simulink model "inverted_pendulum_2D"  (R2016a)
settings: Solver=ode5  SolverMode=SingleTasking  StartTime=0.0  StopTime=Inf  FixedStep=0.01  MaxStep=0.02  RelTol=1e-3
undefined symbols (not defined in the file or in its folder): sl3d_sfuntraj
libraries: vrlib x1
Description:
  | Inverted Pendulum
  | 
  | The vrpend example illustrates the various ways a dynamic model in Simulink(R) can
  | interact with a virtual reality world. It is the model of 2-dimensional inverted pendulum
  | controlled by a PID controller. What distinguishes this model from 'common' inverted
  | pendulum models is visualization and the methods of setting the setpoint. You visualize
  | and interact with a virtual world by using a Trajectory Graph and VR Sink blocks.
  | The Trajectory Graph block allows you to track the history of the pendulum position
  | and change the setpoint. The method for setting the setpoint can be selected in
  | the mask of the Trajectory Graph block. The following methods are available:
  | 
  |   Mouse - Click-and-drag a mouse pointer in the Trajectory Graph 2-D window
  | 
  |   Input Signal - External Trajectory Graph input in this model driven by a random number generator
  | 
  |   VR Sensor - Activates the input from a VRML TouchSensor
  | 
  | When the pointing device in the VRML viewer moves over an active TouchSensor area,
  | the cursor shape changes from an arrow to a hand shape. When the setpoint selection method
  | is set to VRSensor, left mouse button click sets the new setpoint value.
  | 
  | Notice the pseudo orthographic view defined in the associated VRML file. This effect is
  | achieved by creating a viewpoint which is located far from the object of interest with a very narrow
  | view defined by the VRML FieldOfView parameter. An orthographic view is useful for eliminating
  | the panoramic distortion that occurs when using a wide-angle lens. This technique is also
  | known in photography. The fallback of this technique is that locating the viewpoint in a distance
  | makes the standard viewer navigation tricky or difficult in some navigation modes. If you want
  | to navigate around the virtual pendulum bench, we recommend that you switch to some other viewpoint.
settings Model: FPTRunName=Active  ExtModeTrigDuration=100  Creator=The MathWorks, Inc.  LastModifiedBy=USER
settings DataIOCC: LimitDataPoints=on  SaveFormat=Array  SaveOutput=off  SaveTime=off  SignalLoggingName=logsOut
settings OptimizationCC: BlockReduction=off  BooleanDataType=off  ExpressionDepthLimit=2147483647  InitFltsAndDblsToZero=on
settings DebuggingCC: UnderspecifiedInitializationDetection=Classic  MergeDetectMultiDrivingBlocksExec=none  CheckExecutionContextPreStartOutputMsg=on  CheckExecutionContextRuntimeOutputMsg=on  SignalResolutionControl=TryResolveAllWithWarning  MultiTaskDSMMsg=warning  MultiTaskCondExecSysMsg=none  FcnCallInpInsideContextMsg=UseLocalSettings  StateNameClashWarn=warning
settings HardwareCC: ProdBitPerPointer=32  ProdLargestAtomicFloat=None  ProdIntDivRoundTo=Undefined  ProdEndianess=Unspecified  ProdWordSize=32  ProdHWDeviceType=32-bit Generic  TargetUnknown=on
settings ModelReferenceCC: UpdateModelReferenceTargets=IfOutOfDate  PropagateSignalLabelsOutOfModel=off
settings GRTTargetCC: TargetFcnLib=ansi_tfl_tmw.mat  CombineOutputUpdateFcns=off  GRTInterface=on
settings ConfigComp: CovMetricSettings=d  CovModelRefEnable=Off  CovSFcnEnable=off

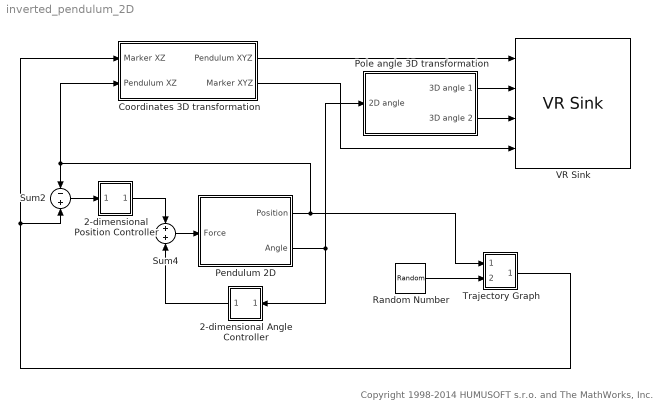
== system inverted_pendulum_2D ==
  note: Copyright 1998-2014 HUMUSOFT s.r.o. and The MathWorks, Inc.
  2-dimensional Angle Controller : Subsystem  mask(PID Controller){P=83.2, I=38.3, D=27.3}
      mask prompts: P "Proportional:"; I "Integral:"; D "Derivative:"
      mask help:
      | Enter expressions for proportional, integral, and derivative terms.
      | P+I/s+Ds
      mask Help: This block implements a PID controller where parameters are entered for the Proportional, Integral and Derivative terms. Unmask this block to see how it works. The derivative term is implemented using a true derivative block.
      mask Display: disp('PID')
  2-dimensional Position Controller : Subsystem  mask(PID Controller){P=-1.681, I=-0.0133, D=-0.325}
      mask prompts: P "Proportional:"; I "Integral:"; D "Derivative:"
      mask help:
      | Enter expressions for proportional, integral, and derivative terms.
      | P+I/s+Ds
      mask Help: This block implements a PID controller where parameters are entered for the Proportional, Integral and Derivative terms. Unmask this block to see how it works. The derivative term is implemented using a true derivative block.
      mask Display: disp('PID')
  Coordinates 3D transformation : Subsystem
  Pendulum 2D : Subsystem  mask(Inverted pendulum){mc=0.5, mp=1, l=0.5, g=9.80665}
      mask prompts: mc "Mass of cart (kg):"; mp "Mass of pendulum (kg):"; l "Distance to pendulum center of mass(m):"; g "Acceleration of gravity (m/s^2):"
      mask help: Look under mask to see dynamics
      mask Help: Nonlinear dynamics of inverted pendulum.
      mask Display: plot([-10 10],[0 0],[-2 -2 2 2],[0 1 1 0],[0 -2],[1 5])
  Pole angle 3D transformation : Subsystem
  Random Number : RandomNumber  Mean=[0 0]  Variance=[5 5]  Seed=[0 5]  SampleTime=3
  Sum2 : Sum  Inputs=-+  SaturateOnIntegerOverflow=on  InputSameDT=on  OutDataTypeStr=Inherit: Same as first input
  Sum4 : Sum  SaturateOnIntegerOverflow=on  InputSameDT=on  OutDataTypeStr=Inherit: Same as first input
  Trajectory Graph : Subsystem  LoadFcn=sl3d_sfuntraj([],[],[],'LoadBlock')  StartFcn=sl3d_sfuntraj([],[],[],'Start')  StopFcn=sl3d_sfuntraj([],[],[],'Stop')  TreatAsAtomicUnit=on  mask(Trajectory scope.){xmin=-10, xmax=10, ymin=-10, ymax=10, Ts=0.2, mode=VR sensor}
      mask prompts: xmin "x-min:"; xmax "x-max:"; ymin "y-min:"; ymax "y-max:"; Ts "Sample time:"; mode "Setpoint mode"
      mask help: Trajectory scope using MATLAB graph window. Enter plotting ranges.
      settings: CopyFcn=sl3d_sfuntraj([],[],[],'CopyBlock')  DeleteFcn=sl3d_sfuntraj([],[],[],'DeleteBlock')  NameChangeFcn=sl3d_sfuntraj([],[],[],'NameChange')
      mask Help: Look at the MATLAB function sl3d_sfuntraj.m to see how this block works.
      mask TypeOptions mode: Mouse | Input signal | VR sensor
      mask Display: plot([.05 .95 .95 .05 .05],[.45 .45 .95 .95 .45], 0.5+cos(0:0.1:2*pi)*0.3,0.7+sin(0:0.1:2*pi)*0.2)
  VR Sink : vrlib/VR Sink  InstantiateOnLoad=on  SampleTime=0.2  ViewEnable=on  RemoteChange=off  RemoteView=off  FieldsWritten=Pendulum.translation.3.1.1.double#Pole1.rotation.4.1.1.double#Pole2.rotation.4.1.1.double#Marker.translation.3.1.1.double  WorldFileName=vrpend.wrl  WorldDescription=Inverted Pendulum  AutoView=on  VideoDimensions=[]  AllowVariableSize=off
  wires:
  Sum4/1 -> Pendulum 2D/1(Force)
  2-dimensional Angle Controller/1(Out_1) -> Sum4/2
  2-dimensional Position Controller/1(Out_1) -> Sum4/1
  Sum2/1 -> 2-dimensional Position Controller/1(In_1)
  Pendulum 2D/2(Angle) -> 2-dimensional Angle Controller/1(In_1), Pole angle 3D transformation/1(2D angle)
  Pendulum 2D/1(Position) -> Sum2/1, Coordinates 3D transformation/2(Pendulum XZ), Trajectory Graph/1(data)
  Trajectory Graph/1(mouse) -> Sum2/2, Coordinates 3D transformation/1(Marker XZ)
  Random Number/1 -> Trajectory Graph/2(setpoint)
  Coordinates 3D transformation/2(Marker XYZ) -> VR Sink/4
  Coordinates 3D transformation/1(Pendulum XYZ) -> VR Sink/1
  Pole angle 3D transformation/1(3D angle 1) -> VR Sink/2
  Pole angle 3D transformation/2(3D angle 2) -> VR Sink/3

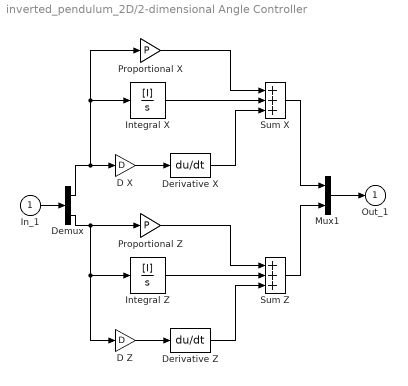
== system inverted_pendulum_2D/2-dimensional Angle Controller ==
  In_1 : Inport
  D X : Gain  Gain=D  SaturateOnIntegerOverflow=on  OutDataTypeStr=Inherit: Same as input  ParamDataTypeStr=Inherit: Same as input
  D Z : Gain  Gain=D  SaturateOnIntegerOverflow=on  OutDataTypeStr=Inherit: Same as input  ParamDataTypeStr=Inherit: Same as input
  Demux : Demux  Outputs=2
  Derivative X : Derivative
  Derivative Z : Derivative
  Integral X : TransferFcn  Numerator=[I]  Denominator=[1 0]
  Integral Z : TransferFcn  Numerator=[I]  Denominator=[1 0]
  Mux1 : Mux  Inputs=2
  Proportional X : Gain  Gain=P  SaturateOnIntegerOverflow=on  OutDataTypeStr=Inherit: Same as input  ParamDataTypeStr=Inherit: Same as input
  Proportional Z : Gain  Gain=P  SaturateOnIntegerOverflow=on  OutDataTypeStr=Inherit: Same as input  ParamDataTypeStr=Inherit: Same as input
  Sum X : Sum  Inputs=+++  SaturateOnIntegerOverflow=on  InputSameDT=on  OutDataTypeStr=Inherit: Same as first input
  Sum Z : Sum  Inputs=+++  SaturateOnIntegerOverflow=on  InputSameDT=on  OutDataTypeStr=Inherit: Same as first input
  Out_1 : Outport  InitialOutput=0
  wires:
  D X/1 -> Derivative X/1
  Derivative X/1 -> Sum X/3
  Integral X/1 -> Sum X/2
  Proportional X/1 -> Sum X/1
  In_1/1 -> Demux/1
  Demux/2 -> Proportional Z/1, Integral Z/1, D Z/1
  Demux/1 -> D X/1, Integral X/1, Proportional X/1
  Sum X/1 -> Mux1/1
  Sum Z/1 -> Mux1/2
  D Z/1 -> Derivative Z/1
  Derivative Z/1 -> Sum Z/3
  Integral Z/1 -> Sum Z/2
  Proportional Z/1 -> Sum Z/1
  Mux1/1 -> Out_1/1

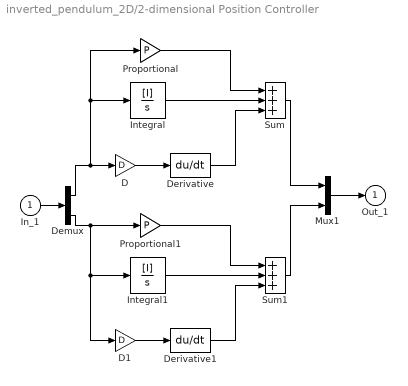
== system inverted_pendulum_2D/2-dimensional Position Controller ==
  In_1 : Inport
  D : Gain  Gain=D  SaturateOnIntegerOverflow=on  OutDataTypeStr=Inherit: Same as input  ParamDataTypeStr=Inherit: Same as input
  D1 : Gain  Gain=D  SaturateOnIntegerOverflow=on  OutDataTypeStr=Inherit: Same as input  ParamDataTypeStr=Inherit: Same as input
  Demux : Demux  Outputs=2
  Derivative : Derivative
  Derivative1 : Derivative
  Integral : TransferFcn  Numerator=[I]  Denominator=[1 0]
  Integral1 : TransferFcn  Numerator=[I]  Denominator=[1 0]
  Mux1 : Mux  Inputs=2
  Proportional : Gain  Gain=P  SaturateOnIntegerOverflow=on  OutDataTypeStr=Inherit: Same as input  ParamDataTypeStr=Inherit: Same as input
  Proportional1 : Gain  Gain=P  SaturateOnIntegerOverflow=on  OutDataTypeStr=Inherit: Same as input  ParamDataTypeStr=Inherit: Same as input
  Sum : Sum  Inputs=+++  SaturateOnIntegerOverflow=on  InputSameDT=on  OutDataTypeStr=Inherit: Same as first input
  Sum1 : Sum  Inputs=+++  SaturateOnIntegerOverflow=on  InputSameDT=on  OutDataTypeStr=Inherit: Same as first input
  Out_1 : Outport  InitialOutput=0
  wires:
  Mux1/1 -> Out_1/1
  Proportional1/1 -> Sum1/1
  Integral1/1 -> Sum1/2
  Derivative1/1 -> Sum1/3
  D1/1 -> Derivative1/1
  Sum1/1 -> Mux1/2
  Sum/1 -> Mux1/1
  Demux/1 -> Proportional/1, Integral/1, D/1
  Demux/2 -> D1/1, Integral1/1, Proportional1/1
  In_1/1 -> Demux/1
  Proportional/1 -> Sum/1
  Integral/1 -> Sum/2
  Derivative/1 -> Sum/3
  D/1 -> Derivative/1

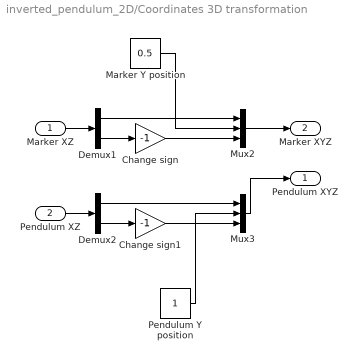
== system inverted_pendulum_2D/Coordinates 3D transformation ==
  Marker XZ : Inport
  Pendulum XZ : Inport  Port=2
  Change sign : Gain  Gain=-1
  Change sign1 : Gain  Gain=-1
  Demux1 : Demux  Outputs=2
  Demux2 : Demux  Outputs=2
  Marker Y position : Constant  Value=0.5
  Mux2 : Mux  Inputs=3
  Mux3 : Mux  Inputs=3
  Pendulum Y position : Constant
  Pendulum XYZ : Outport
  Marker XYZ : Outport  Port=2
  wires:
  Marker XZ/1 -> Demux1/1
  Pendulum XZ/1 -> Demux2/1
  Pendulum Y position/1 -> Mux3/2
  Marker Y position/1 -> Mux2/2
  Mux2/1 -> Marker XYZ/1
  Mux3/1 -> Pendulum XYZ/1
  Demux1/1 -> Mux2/1
  Demux1/2 -> Change sign/1
  Demux2/2 -> Change sign1/1
  Change sign/1 -> Mux2/3
  Demux2/1 -> Mux3/1
  Change sign1/1 -> Mux3/3

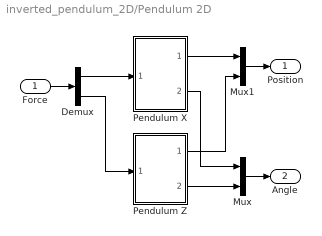
== system inverted_pendulum_2D/Pendulum 2D ==
  Force : Inport
  Demux : Demux  Outputs=2
  Mux : Mux  Inputs=2
  Mux1 : Mux  Inputs=2
  Pendulum X : Subsystem  mask(Inverted pendulum){mc=mc, mp=mp, l=l, g=g}
      mask prompts: mc "Mass of cart (kg):"; mp "Mass of pendulum (kg):"; l "Distance to pendulum center of mass(m):"; g "Acceleration of gravity (m/s^2):"
      mask help: Look under mask to see dynamics
      mask Help: Nonlinear dynamics of inverted pendulum.
  Pendulum Z : Subsystem  mask(Inverted pendulum){mc=mc, mp=mp, l=l, g=g}
      mask prompts: mc "Mass of cart (kg):"; mp "Mass of pendulum (kg):"; l "Distance to pendulum center of mass(m):"; g "Acceleration of gravity (m/s^2):"
      mask help: Look under mask to see dynamics
      mask Help: Nonlinear dynamics of inverted pendulum.
  Position : Outport
  Angle : Outport  Port=2
  wires:
  Pendulum X/1(Position) -> Mux1/1
  Pendulum Z/1(Position) -> Mux1/2
  Pendulum Z/2(Angle) -> Mux/2
  Pendulum X/2(Angle) -> Mux/1
  Demux/1 -> Pendulum X/1(Force)
  Demux/2 -> Pendulum Z/1(Force)
  Mux1/1 -> Position/1
  Force/1 -> Demux/1
  Mux/1 -> Angle/1

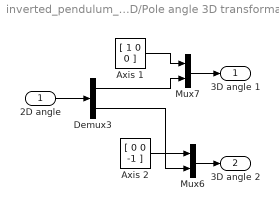
== system inverted_pendulum_2D/Pole angle 3D transformation ==
  2D angle : Inport
  Axis 1 : Constant  Value=[ 1 0 0 ]
  Axis 2 : Constant  Value=[ 0 0 -1 ]
  Demux3 : Demux  Outputs=2
  Mux6 : Mux  Inputs=2
  Mux7 : Mux  Inputs=2
  3D angle 1 : Outport
  3D angle 2 : Outport  Port=2
  wires:
  Axis 1/1 -> Mux7/1
  Axis 2/1 -> Mux6/1
  2D angle/1 -> Demux3/1
  Mux7/1 -> 3D angle 1/1
  Demux3/1 -> Mux7/2
  Demux3/2 -> Mux6/2
  Mux6/1 -> 3D angle 2/1

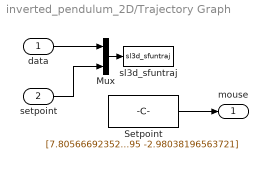
== system inverted_pendulum_2D/Trajectory Graph ==
  data : Inport
  setpoint : Inport  Port=2
  Mux : Mux  Inputs=2
  Setpoint : Constant  Priority=20  Value=[7.80566692352295 -2.98038196563721]  SampleTime=Ts
  sl3d_sfuntraj : S-Function  Priority=10  FunctionName=sl3d_sfuntraj  Parameters=[xmin xmax ymin ymax], Ts, mode  SFunctionDeploymentMode=off  EnableBusSupport=off
  mouse : Outport
  wires:
  setpoint/1 -> Mux/2
  data/1 -> Mux/1
  Mux/1 -> sl3d_sfuntraj/1
  Setpoint/1 -> mouse/1

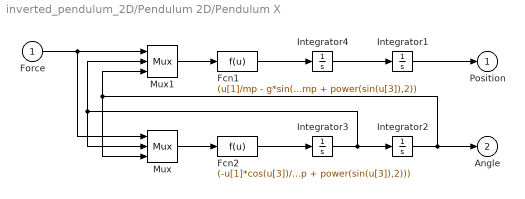
== system inverted_pendulum_2D/Pendulum 2D/Pendulum X ==
  Force : Inport
  Fcn1 : Fcn  Expr=(u[1]/mp - g*sin(u[3])*cos(u[3]) + l*power(u[2],2)*sin(u[3]))/(mc/mp + power(sin(u[3]),2))
  Fcn2 : Fcn  Expr=(-u[1]*cos(u[3])/mp + (mc+mp)*g*sin(u[3])/mp - l*power(u[2],2)*sin(u[3])*cos(u[3]))/(l*(mc/mp + power(sin(u[3]),2)))
  Integrator1 : Integrator  UpperSaturationLimit=Inf  LowerSaturationLimit=-Inf  ZeroCross=off
  Integrator2 : Integrator  LimitOutput=on  UpperSaturationLimit=pi/2  LowerSaturationLimit=-pi/2  ZeroCross=off
  Integrator3 : Integrator  UpperSaturationLimit=Inf  LowerSaturationLimit=-Inf  ZeroCross=off
  Integrator4 : Integrator  UpperSaturationLimit=Inf  LowerSaturationLimit=-Inf  ZeroCross=off
  Mux : Mux  Inputs=3
  Mux1 : Mux  Inputs=3
  Position : Outport  InitialOutput=0
  Angle : Outport  Port=2  InitialOutput=0
  wires:
  Integrator2/1 -> Mux/3, Mux1/3, Angle/1
  Integrator3/1 -> Mux/2, Mux1/2, Integrator2/1
  Force/1 -> Mux/1, Mux1/1
  Integrator4/1 -> Integrator1/1
  Fcn1/1 -> Integrator4/1
  Mux1/1 -> Fcn1/1
  Mux/1 -> Fcn2/1
  Fcn2/1 -> Integrator3/1
  Integrator1/1 -> Position/1

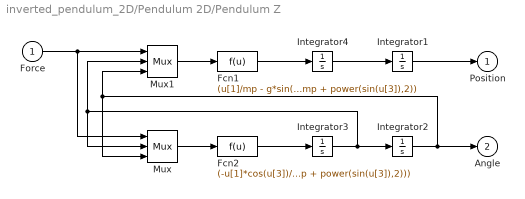
== system inverted_pendulum_2D/Pendulum 2D/Pendulum Z ==
  Force : Inport
  Fcn1 : Fcn  Expr=(u[1]/mp - g*sin(u[3])*cos(u[3]) + l*power(u[2],2)*sin(u[3]))/(mc/mp + power(sin(u[3]),2))
  Fcn2 : Fcn  Expr=(-u[1]*cos(u[3])/mp + (mc+mp)*g*sin(u[3])/mp - l*power(u[2],2)*sin(u[3])*cos(u[3]))/(l*(mc/mp + power(sin(u[3]),2)))
  Integrator1 : Integrator  UpperSaturationLimit=Inf  LowerSaturationLimit=-Inf  ZeroCross=off
  Integrator2 : Integrator  LimitOutput=on  UpperSaturationLimit=pi/2  LowerSaturationLimit=-pi/2  ZeroCross=off
  Integrator3 : Integrator  UpperSaturationLimit=Inf  LowerSaturationLimit=-Inf  ZeroCross=off
  Integrator4 : Integrator  UpperSaturationLimit=Inf  LowerSaturationLimit=-Inf  ZeroCross=off
  Mux : Mux  Inputs=3
  Mux1 : Mux  Inputs=3
  Position : Outport  InitialOutput=0
  Angle : Outport  Port=2  InitialOutput=0
  wires:
  Integrator1/1 -> Position/1
  Fcn2/1 -> Integrator3/1
  Mux/1 -> Fcn2/1
  Mux1/1 -> Fcn1/1
  Fcn1/1 -> Integrator4/1
  Integrator4/1 -> Integrator1/1
  Force/1 -> Mux1/1, Mux/1
  Integrator3/1 -> Integrator2/1, Mux1/2, Mux/2
  Integrator2/1 -> Angle/1, Mux1/3, Mux/3
